simulink model "Events6"  (Simulink 5.0)
settings: Solver=ode45  StartTime=0.0  StopTime=10.0  RelTol=1e-3
settings Model: Creator=scaife  LastModifiedBy=scaife  ExtModeAutoUpdateStatusClock=off

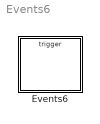
== system Events6 ==
  Events6 : Stateflow chart

== stateflow chart Events6 ==
  state T1 [parallel]
    state A
    state B
    (default) -> A
    A -> B : E/F
    B -> A : E/G
  state T2 [parallel]
    state C
    state D
    state E
    (default) -> C
    C -> D : F
    D -> C : G
    D -> E : F
    E -> D : G
  events: E input EITHER_EDGE_EVENT; F local EITHER_EDGE_EVENT; G local EITHER_EDGE_EVENT
